simulink subsystem "DCDriver_Ideal"  (R2023b)
settings: Solver=VariableStepAuto  StartTime=0.0  StopTime=10.0  RelTol=1e-3
libraries: fl_lib x2, nesl_utility x1
settings Model: DataDictionary=neck_mk3.sldd  EnableAccessToBaseWorkspace=off  Creator=upattacini  LastModifiedBy=upattacini

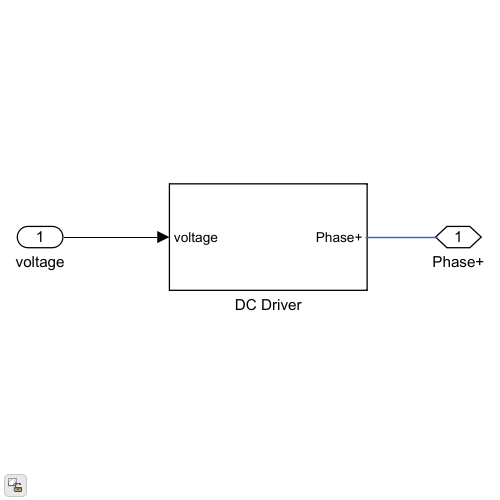
[thumbnail: Simulink's stored preview of the top-level diagram]
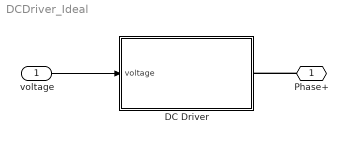
== system DCDriver_Ideal ==
  voltage : Inport  Unit=%  PortDimensions=1
  DC Driver : Subsystem  mask{Supply_Vcc=12}
      mask prompts: Supply_Vcc "Supply Voltage (V)"
  Phase+ : PMIOPort  Side=Right
  wires:
  voltage/1 -> DC Driver/1(voltage)
  connections:
  Phase+/RConn1 -- DC Driver/RConn1

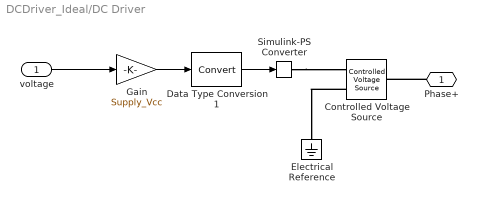
== system DCDriver_Ideal/DC Driver ==
  voltage : Inport
  Controlled Voltage Source : fl_lib/Electrical/Electrical Sources/Controlled Voltage Source
  Data Type Conversion1 : DataTypeConversion  SaturateOnIntegerOverflow=off  RndMeth=Floor
  Electrical Reference : fl_lib/Electrical/Electrical Elements/Electrical Reference
  Gain : Gain  Gain=Supply_Vcc
  Simulink-PS Converter : nesl_utility/Simulink-PS Converter  PhysicalDomain=network_engine_domain  SubClassName=ps_input  LeftPortType=input  RightPortType=output  PseudoPeriodic=off  Frequencies=[]  NoiseDistribution=none  NoiseParameters=[]  Unit=V  AffineConversion=off  FilteringAndDerivatives=provide  SimscapeFilterOrder=1  InputFilterTimeConstant=0.001  UdotUserProvided=0
  Phase+ : PMIOPort  Side=Right
  wires:
  voltage/1 -> Gain/1
  Data Type Conversion1/1 -> Simulink-PS Converter/1
  Gain/1 -> Data Type Conversion1/1
  connections:
  Controlled Voltage Source/RConn2 -- Electrical Reference/LConn1
  Phase+/RConn1 -- Controlled Voltage Source/LConn1
  Simulink-PS Converter/RConn1 -- Controlled Voltage Source/RConn1
